simulink model "Space_vector_pwm_deneme"  (R2018a)
settings: Solver=VariableStepDiscrete  StartTime=0.0  StopTime=10  RelTol=1e-3
libraries: powerlib x4, electricdrivelib x1
settings Model: Creator=bulbu  LastModifiedBy=bulbu

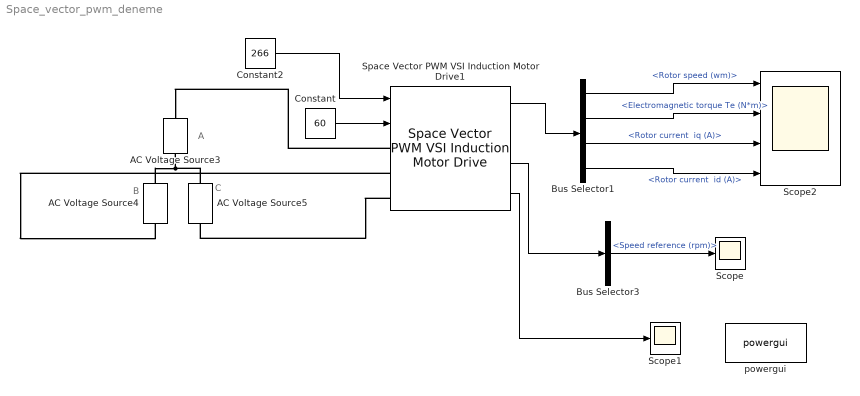
== system Space_vector_pwm_deneme ==
  note: C
  note: A
  note: B
  AC Voltage Source3 : powerlib/Electrical Sources/AC Voltage Source  Amplitude=326.6  Phase=0  Frequency=50  SampleTime=0  Measurements=None  BusType=swing  Pref=10e3  Qref=0  Qmin=-inf  Qmax=+inf
  AC Voltage Source4 : powerlib/Electrical Sources/AC Voltage Source  Amplitude=326.6  Phase=120  Frequency=50  SampleTime=0  Measurements=None  BusType=swing  Pref=10e3  Qref=0  Qmin=-inf  Qmax=+inf
  AC Voltage Source5 : powerlib/Electrical Sources/AC Voltage Source  Amplitude=326.6  Phase=240  Frequency=50  SampleTime=0  Measurements=None  BusType=swing  Pref=10e3  Qref=0  Qmin=-inf  Qmax=+inf
  Bus Selector1 : BusSelector  OutputSignals="Mechanical.Rotor speed (wm),Mechanical.Electromagnetic torque Te (N*m),Rotor measurements.Rotor current  iq (A),Rotor measurements.Rotor current  id (A)"
  Bus Selector3 : BusSelector  OutputSignals=Speed reference (rpm)
  Constant : Constant  Value=60
  Constant2 : Constant  Value=266
  Scope : Scope
  Scope1 : Scope
  Scope2 : Scope  NumInputPorts=4
  Space Vector PWM VSI Induction Motor Drive1 : electricdrivelib/AC drives/Space Vector PWM VSI Induction Motor Drive  ReferenceFrame=Stationary  IterativeDiscreteModel=Trapezoidal non iterative  Pn=80000  Vn=320  fn=50  Rs=0.435  Lls=0.002  Lms=69.31e-3  Rr=0.816  Llr=0.002  ia=0  pha=0  ib=0  phb=0  ic=0  phc=0  J=0.089  Friction=0.005  p=2  slip=1  thdeg=0  Rsnb_rec=10e3  Csnb_rec=20e-9  Ron_rec=1e-3  Vf_rec=1.3  cap_bus=3400e-6  Rbrake=8  fbrake=4000  activationVoltage=340  shutdownVoltage=320  deviceType=IGBT / Diodes  Ron_inv=1e-3  Vf_inv=1.2  Vfd_inv=1.2  Tf=1e-6  Tt=2e-6  Tf_GTO=1e-6  Tt_GTO=2e-6  Rsnb_inv=500  Csnb_inv=10e-9  Acc=1800  Dec=-1800  kp_sc=200  ki_sc=2000  fc_sc=100  Tsc=100e-6  ctrl_sat_min=-30  ctrl_sat_max=30  ctrl_f_min=0.05  ctrl_f_max=120  ctrl_v_min=10  ctrl_v_max=180  vh_ratio=6  zc_time=0.4  car_freq=20000  fc_bus=50  Tvect=20e-6  baseSampleTime=2e-06  outputBusMode=Multiple output buses  busLabels=off  MechanicalLoad=Torque Tm  modelDetailLevel=Detailed  driveType=AC2  AverageValue=off
      settings: SourceProductName=Simscape Power Systems  SourceProductBaseCode=PS
  powergui : powerlib/powergui  Priority=1  SimulationMode=Discrete  SampleTime=1e-5  frequency=60  Iterations=50  frequencyindice=0  Pbase=100e6  ErrMax=1e-4  UnitsV=kV  UnitsW=MW  buscounter=0  FunctionMessages=off  echomessages=off  EnableUseOfTLC=off  CurrentSourceSwitches=off  DisableSnubberDevices=off  DisableRonSwitches=off  DisableVfSwitches=off  DisplayEquations=off  SolverType=Tustin/Backward Euler (TBE)  Interpol=off  ExternalGateDelay=off  methode=off  Ts=100  x0status=blocks  SPID=on  SwTol=0  HookPort=off  RestoreLinks=warning  ResistiveCurrentMeasurement=off  Frange=[0:2:500]  Ylog=off  Xlog=on  ShowGrid=off  save=off  variable=ZData  structure=0  ZoomFFT=off  StartTime=0.0  cycles=1  DisplayStyle=1  fundamental=60  FreqAxis=off  MaxFrequency=1000  frequencyindicesteady=1  RmsSteady=1  display=off
  wires:
  Space Vector PWM VSI Induction Motor Drive1/1 -> Bus Selector1/1
  Bus Selector1/1 -> Scope2/1  "<Rotor speed (wm)>"
  Bus Selector1/2 -> Scope2/2  "<Electromagnetic torque Te (N*m)>"
  Bus Selector1/3 -> Scope2/3  "<Rotor current  iq (A)>"
  Bus Selector1/4 -> Scope2/4  "<Rotor current  id (A)>"
  Space Vector PWM VSI Induction Motor Drive1/3 -> Bus Selector3/1
  Constant2/1 -> Space Vector PWM VSI Induction Motor Drive1/1
  Bus Selector3/1 -> Scope/1  "<Speed reference (rpm)>"
  Space Vector PWM VSI Induction Motor Drive1/4 -> Scope1/1
  Constant/1 -> Space Vector PWM VSI Induction Motor Drive1/2
  connections:
  AC Voltage Source4/LConn1 -- AC Voltage Source3/LConn1 -- AC Voltage Source5/LConn1
  Space Vector PWM VSI Induction Motor Drive1/LConn1 -- AC Voltage Source3/RConn1
  Space Vector PWM VSI Induction Motor Drive1/LConn3 -- AC Voltage Source5/RConn1
  Space Vector PWM VSI Induction Motor Drive1/LConn2 -- AC Voltage Source4/RConn1
